simulink model "Pokus07_Display"  (Simulink 8.1)
settings: Solver=ode45  StartTime=0.0  StopTime=10.0  RelTol=1e-3
undefined symbols (not defined in the file): A, ARROW_DOWN, ARROW_LEFT, ARROW_RIGHT, ARROW_UP, ASTERISK, B, BACKSLASH, C, COLON, COMMA, CROSS, CURSOR, D, DOT, ending_column_index, ending_row_index, EQUAL, EXCLAMATION_MARK, F, framebuffer, G, GREATER_THAN, H, HEIGHT, hot, I, J, K, L, LEFT_PARENTHESES, LESS_THAN, M, MINUS, N, O, P, PERCENT, PLUS, POS_X, POS_Y, Q, QUESTION_MARK, QUOTE, R, RECTANGLE, RIGHT_PARENTHESES, S, SEMICOLON, SHARP, SLASH, SPACE, starting_column_index, starting_row_index, T, U, UNDERSCORE, V, W, WIDTH ... (+6)
libraries: dspmtrx3 x197, Common_Library x69, commutil2 x53, simulink_extras x1, dspsnks4 x1
(part 4 of 6)

== system Pokus07_Display/Character_Table/Characters(ARROW_DOWN..RECTANGLE)/Char_ARROW_LEFT ==
  Byte_01 : Constant  Value=char(2, ARROW_LEFT)  OutDataTypeStr=uint8
  Byte_02 : Constant  Value=char(3, ARROW_LEFT)  OutDataTypeStr=uint8
  Byte_03 : Constant  Value=char(4, ARROW_LEFT)  OutDataTypeStr=uint8
  Byte_04 : Constant  Value=char(5, ARROW_LEFT)  OutDataTypeStr=uint8
  Byte_05 : Constant  Value=char(6, ARROW_LEFT)  OutDataTypeStr=uint8
  Byte_06 : Constant  Value=char(7, ARROW_LEFT)  OutDataTypeStr=uint8
  Byte_07 : Constant  Value=char(8, ARROW_LEFT)  OutDataTypeStr=uint8
  Byte_1 : Constant  Value=char(1, ARROW_LEFT)  OutDataTypeStr=uint8
  Column_1(1B) : Outport
  Column_2(1B) : Outport  Port=2
  Column_3(1B) : Outport  Port=3
  Column_4(1B) : Outport  Port=4
  Column_5(1B) : Outport  Port=5
  Column_6(1B) : Outport  Port=6
  Column_7(1B) : Outport  Port=7
  Column_8(1B) : Outport  Port=8
  wires:
  Byte_05/1 -> Column_6(1B)/1
  Byte_04/1 -> Column_5(1B)/1
  Byte_01/1 -> Column_2(1B)/1
  Byte_07/1 -> Column_8(1B)/1
  Byte_03/1 -> Column_4(1B)/1
  Byte_06/1 -> Column_7(1B)/1
  Byte_1/1 -> Column_1(1B)/1
  Byte_02/1 -> Column_3(1B)/1

== system Pokus07_Display/Character_Table/Characters(ARROW_DOWN..RECTANGLE)/Char_ARROW_RIGHT ==
  Byte_01 : Constant  Value=char(2, ARROW_RIGHT)  OutDataTypeStr=uint8
  Byte_02 : Constant  Value=char(3, ARROW_RIGHT)  OutDataTypeStr=uint8
  Byte_03 : Constant  Value=char(4, ARROW_RIGHT)  OutDataTypeStr=uint8
  Byte_04 : Constant  Value=char(5, ARROW_RIGHT)  OutDataTypeStr=uint8
  Byte_05 : Constant  Value=char(6, ARROW_RIGHT)  OutDataTypeStr=uint8
  Byte_06 : Constant  Value=char(7, ARROW_RIGHT)  OutDataTypeStr=uint8
  Byte_07 : Constant  Value=char(8, ARROW_RIGHT)  OutDataTypeStr=uint8
  Byte_1 : Constant  Value=char(1, ARROW_RIGHT)  OutDataTypeStr=uint8
  Column_1(1B) : Outport
  Column_2(1B) : Outport  Port=2
  Column_3(1B) : Outport  Port=3
  Column_4(1B) : Outport  Port=4
  Column_5(1B) : Outport  Port=5
  Column_6(1B) : Outport  Port=6
  Column_7(1B) : Outport  Port=7
  Column_8(1B) : Outport  Port=8
  wires:
  Byte_05/1 -> Column_6(1B)/1
  Byte_04/1 -> Column_5(1B)/1
  Byte_01/1 -> Column_2(1B)/1
  Byte_07/1 -> Column_8(1B)/1
  Byte_03/1 -> Column_4(1B)/1
  Byte_06/1 -> Column_7(1B)/1
  Byte_1/1 -> Column_1(1B)/1
  Byte_02/1 -> Column_3(1B)/1

== system Pokus07_Display/Character_Table/Characters(ARROW_DOWN..RECTANGLE)/Char_COMMA ==
  Byte_01 : Constant  Value=char(2, COMMA)  OutDataTypeStr=uint8
  Byte_02 : Constant  Value=char(3, COMMA)  OutDataTypeStr=uint8
  Byte_03 : Constant  Value=char(4, COMMA)  OutDataTypeStr=uint8
  Byte_04 : Constant  Value=char(5, COMMA)  OutDataTypeStr=uint8
  Byte_05 : Constant  Value=char(6, COMMA)  OutDataTypeStr=uint8
  Byte_06 : Constant  Value=char(7, COMMA)  OutDataTypeStr=uint8
  Byte_07 : Constant  Value=char(8, COMMA)  OutDataTypeStr=uint8
  Byte_1 : Constant  Value=char(1, COMMA)  OutDataTypeStr=uint8
  Column_1(1B) : Outport
  Column_2(1B) : Outport  Port=2
  Column_3(1B) : Outport  Port=3
  Column_4(1B) : Outport  Port=4
  Column_5(1B) : Outport  Port=5
  Column_6(1B) : Outport  Port=6
  Column_7(1B) : Outport  Port=7
  Column_8(1B) : Outport  Port=8
  wires:
  Byte_05/1 -> Column_6(1B)/1
  Byte_04/1 -> Column_5(1B)/1
  Byte_01/1 -> Column_2(1B)/1
  Byte_07/1 -> Column_8(1B)/1
  Byte_03/1 -> Column_4(1B)/1
  Byte_06/1 -> Column_7(1B)/1
  Byte_1/1 -> Column_1(1B)/1
  Byte_02/1 -> Column_3(1B)/1

== system Pokus07_Display/Character_Table/Characters(ARROW_DOWN..RECTANGLE)/Char_CURSOR ==
  Byte_01 : Constant  Value=char(2, CURSOR)  OutDataTypeStr=uint8
  Byte_02 : Constant  Value=char(3, CURSOR)  OutDataTypeStr=uint8
  Byte_03 : Constant  Value=char(4, CURSOR)  OutDataTypeStr=uint8
  Byte_04 : Constant  Value=char(5, CURSOR)  OutDataTypeStr=uint8
  Byte_05 : Constant  Value=char(6, CURSOR)  OutDataTypeStr=uint8
  Byte_06 : Constant  Value=char(7, CURSOR)  OutDataTypeStr=uint8
  Byte_07 : Constant  Value=char(8, CURSOR)  OutDataTypeStr=uint8
  Byte_1 : Constant  Value=char(1, CURSOR)  OutDataTypeStr=uint8
  Column_1(1B) : Outport
  Column_2(1B) : Outport  Port=2
  Column_3(1B) : Outport  Port=3
  Column_4(1B) : Outport  Port=4
  Column_5(1B) : Outport  Port=5
  Column_6(1B) : Outport  Port=6
  Column_7(1B) : Outport  Port=7
  Column_8(1B) : Outport  Port=8
  wires:
  Byte_05/1 -> Column_6(1B)/1
  Byte_04/1 -> Column_5(1B)/1
  Byte_01/1 -> Column_2(1B)/1
  Byte_07/1 -> Column_8(1B)/1
  Byte_03/1 -> Column_4(1B)/1
  Byte_06/1 -> Column_7(1B)/1
  Byte_1/1 -> Column_1(1B)/1
  Byte_02/1 -> Column_3(1B)/1

== system Pokus07_Display/Character_Table/Characters(ARROW_DOWN..RECTANGLE)/Char_DOT ==
  Byte_01 : Constant  Value=char(2, DOT)  OutDataTypeStr=uint8
  Byte_02 : Constant  Value=char(3, DOT)  OutDataTypeStr=uint8
  Byte_03 : Constant  Value=char(4, DOT)  OutDataTypeStr=uint8
  Byte_04 : Constant  Value=char(5, DOT)  OutDataTypeStr=uint8
  Byte_05 : Constant  Value=char(6, DOT)  OutDataTypeStr=uint8
  Byte_06 : Constant  Value=char(7, DOT)  OutDataTypeStr=uint8
  Byte_07 : Constant  Value=char(8, DOT)  OutDataTypeStr=uint8
  Byte_1 : Constant  Value=char(1, DOT)  OutDataTypeStr=uint8
  Column_1(1B) : Outport
  Column_2(1B) : Outport  Port=2
  Column_3(1B) : Outport  Port=3
  Column_4(1B) : Outport  Port=4
  Column_5(1B) : Outport  Port=5
  Column_6(1B) : Outport  Port=6
  Column_7(1B) : Outport  Port=7
  Column_8(1B) : Outport  Port=8
  wires:
  Byte_05/1 -> Column_6(1B)/1
  Byte_04/1 -> Column_5(1B)/1
  Byte_01/1 -> Column_2(1B)/1
  Byte_07/1 -> Column_8(1B)/1
  Byte_03/1 -> Column_4(1B)/1
  Byte_06/1 -> Column_7(1B)/1
  Byte_1/1 -> Column_1(1B)/1
  Byte_02/1 -> Column_3(1B)/1

== system Pokus07_Display/Character_Table/Characters(ARROW_DOWN..RECTANGLE)/Char_EXCLAMATION_MARK ==
  Byte_01 : Constant  Value=char(2, EXCLAMATION_MARK)  OutDataTypeStr=uint8
  Byte_02 : Constant  Value=char(3, EXCLAMATION_MARK)  OutDataTypeStr=uint8
  Byte_03 : Constant  Value=char(4, EXCLAMATION_MARK)  OutDataTypeStr=uint8
  Byte_04 : Constant  Value=char(5, EXCLAMATION_MARK)  OutDataTypeStr=uint8
  Byte_05 : Constant  Value=char(6, EXCLAMATION_MARK)  OutDataTypeStr=uint8
  Byte_06 : Constant  Value=char(7, EXCLAMATION_MARK)  OutDataTypeStr=uint8
  Byte_07 : Constant  Value=char(8, EXCLAMATION_MARK)  OutDataTypeStr=uint8
  Byte_1 : Constant  Value=char(1, EXCLAMATION_MARK)  OutDataTypeStr=uint8
  Column_1(1B) : Outport
  Column_2(1B) : Outport  Port=2
  Column_3(1B) : Outport  Port=3
  Column_4(1B) : Outport  Port=4
  Column_5(1B) : Outport  Port=5
  Column_6(1B) : Outport  Port=6
  Column_7(1B) : Outport  Port=7
  Column_8(1B) : Outport  Port=8
  wires:
  Byte_05/1 -> Column_6(1B)/1
  Byte_04/1 -> Column_5(1B)/1
  Byte_01/1 -> Column_2(1B)/1
  Byte_07/1 -> Column_8(1B)/1
  Byte_03/1 -> Column_4(1B)/1
  Byte_06/1 -> Column_7(1B)/1
  Byte_1/1 -> Column_1(1B)/1
  Byte_02/1 -> Column_3(1B)/1

== system Pokus07_Display/Character_Table/Characters(ARROW_DOWN..RECTANGLE)/Char_LEFT_PARENTHESES ==
  Byte_01 : Constant  Value=char(2, LEFT_PARENTHESES)  OutDataTypeStr=uint8
  Byte_02 : Constant  Value=char(3, LEFT_PARENTHESES)  OutDataTypeStr=uint8
  Byte_03 : Constant  Value=char(4, LEFT_PARENTHESES)  OutDataTypeStr=uint8
  Byte_04 : Constant  Value=char(5, LEFT_PARENTHESES)  OutDataTypeStr=uint8
  Byte_05 : Constant  Value=char(6, LEFT_PARENTHESES)  OutDataTypeStr=uint8
  Byte_06 : Constant  Value=char(7, LEFT_PARENTHESES)  OutDataTypeStr=uint8
  Byte_07 : Constant  Value=char(8, LEFT_PARENTHESES)  OutDataTypeStr=uint8
  Byte_1 : Constant  Value=char(1, LEFT_PARENTHESES)  OutDataTypeStr=uint8
  Column_1(1B) : Outport
  Column_2(1B) : Outport  Port=2
  Column_3(1B) : Outport  Port=3
  Column_4(1B) : Outport  Port=4
  Column_5(1B) : Outport  Port=5
  Column_6(1B) : Outport  Port=6
  Column_7(1B) : Outport  Port=7
  Column_8(1B) : Outport  Port=8
  wires:
  Byte_05/1 -> Column_6(1B)/1
  Byte_04/1 -> Column_5(1B)/1
  Byte_01/1 -> Column_2(1B)/1
  Byte_07/1 -> Column_8(1B)/1
  Byte_03/1 -> Column_4(1B)/1
  Byte_06/1 -> Column_7(1B)/1
  Byte_1/1 -> Column_1(1B)/1
  Byte_02/1 -> Column_3(1B)/1

== system Pokus07_Display/Character_Table/Characters(ARROW_DOWN..RECTANGLE)/Char_PERCENT ==
  Byte_01 : Constant  Value=char(2, PERCENT)  OutDataTypeStr=uint8
  Byte_02 : Constant  Value=char(3, PERCENT)  OutDataTypeStr=uint8
  Byte_03 : Constant  Value=char(4, PERCENT)  OutDataTypeStr=uint8
  Byte_04 : Constant  Value=char(5, PERCENT)  OutDataTypeStr=uint8
  Byte_05 : Constant  Value=char(6, PERCENT)  OutDataTypeStr=uint8
  Byte_06 : Constant  Value=char(7, PERCENT)  OutDataTypeStr=uint8
  Byte_07 : Constant  Value=char(8, PERCENT)  OutDataTypeStr=uint8
  Byte_1 : Constant  Value=char(1, PERCENT)  OutDataTypeStr=uint8
  Column_1(1B) : Outport
  Column_2(1B) : Outport  Port=2
  Column_3(1B) : Outport  Port=3
  Column_4(1B) : Outport  Port=4
  Column_5(1B) : Outport  Port=5
  Column_6(1B) : Outport  Port=6
  Column_7(1B) : Outport  Port=7
  Column_8(1B) : Outport  Port=8
  wires:
  Byte_05/1 -> Column_6(1B)/1
  Byte_04/1 -> Column_5(1B)/1
  Byte_01/1 -> Column_2(1B)/1
  Byte_07/1 -> Column_8(1B)/1
  Byte_03/1 -> Column_4(1B)/1
  Byte_06/1 -> Column_7(1B)/1
  Byte_1/1 -> Column_1(1B)/1
  Byte_02/1 -> Column_3(1B)/1

== system Pokus07_Display/Character_Table/Characters(ARROW_DOWN..RECTANGLE)/Char_QUESTION_MARK ==
  Byte_01 : Constant  Value=char(2, QUESTION_MARK)  OutDataTypeStr=uint8
  Byte_02 : Constant  Value=char(3, QUESTION_MARK)  OutDataTypeStr=uint8
  Byte_03 : Constant  Value=char(4, QUESTION_MARK)  OutDataTypeStr=uint8
  Byte_04 : Constant  Value=char(5, QUESTION_MARK)  OutDataTypeStr=uint8
  Byte_05 : Constant  Value=char(6, QUESTION_MARK)  OutDataTypeStr=uint8
  Byte_06 : Constant  Value=char(7, QUESTION_MARK)  OutDataTypeStr=uint8
  Byte_07 : Constant  Value=char(8, QUESTION_MARK)  OutDataTypeStr=uint8
  Byte_1 : Constant  Value=char(1, QUESTION_MARK)  OutDataTypeStr=uint8
  Column_1(1B) : Outport
  Column_2(1B) : Outport  Port=2
  Column_3(1B) : Outport  Port=3
  Column_4(1B) : Outport  Port=4
  Column_5(1B) : Outport  Port=5
  Column_6(1B) : Outport  Port=6
  Column_7(1B) : Outport  Port=7
  Column_8(1B) : Outport  Port=8
  wires:
  Byte_05/1 -> Column_6(1B)/1
  Byte_04/1 -> Column_5(1B)/1
  Byte_01/1 -> Column_2(1B)/1
  Byte_07/1 -> Column_8(1B)/1
  Byte_03/1 -> Column_4(1B)/1
  Byte_06/1 -> Column_7(1B)/1
  Byte_1/1 -> Column_1(1B)/1
  Byte_02/1 -> Column_3(1B)/1

== system Pokus07_Display/Character_Table/Characters(ARROW_DOWN..RECTANGLE)/Char_QUOTE ==
  Byte_01 : Constant  Value=char(2, QUOTE)  OutDataTypeStr=uint8
  Byte_02 : Constant  Value=char(3, QUOTE)  OutDataTypeStr=uint8
  Byte_03 : Constant  Value=char(4, QUOTE)  OutDataTypeStr=uint8
  Byte_04 : Constant  Value=char(5, QUOTE)  OutDataTypeStr=uint8
  Byte_05 : Constant  Value=char(6, QUOTE)  OutDataTypeStr=uint8
  Byte_06 : Constant  Value=char(7, QUOTE)  OutDataTypeStr=uint8
  Byte_07 : Constant  Value=char(8, QUOTE)  OutDataTypeStr=uint8
  Byte_1 : Constant  Value=char(1, QUOTE)  OutDataTypeStr=uint8
  Column_1(1B) : Outport
  Column_2(1B) : Outport  Port=2
  Column_3(1B) : Outport  Port=3
  Column_4(1B) : Outport  Port=4
  Column_5(1B) : Outport  Port=5
  Column_6(1B) : Outport  Port=6
  Column_7(1B) : Outport  Port=7
  Column_8(1B) : Outport  Port=8
  wires:
  Byte_05/1 -> Column_6(1B)/1
  Byte_04/1 -> Column_5(1B)/1
  Byte_01/1 -> Column_2(1B)/1
  Byte_07/1 -> Column_8(1B)/1
  Byte_03/1 -> Column_4(1B)/1
  Byte_06/1 -> Column_7(1B)/1
  Byte_1/1 -> Column_1(1B)/1
  Byte_02/1 -> Column_3(1B)/1

== system Pokus07_Display/Character_Table/Characters(ARROW_DOWN..RECTANGLE)/Char_RECTANGLE ==
  Byte_01 : Constant  Value=char(2, RECTANGLE)  OutDataTypeStr=uint8
  Byte_02 : Constant  Value=char(3, RECTANGLE)  OutDataTypeStr=uint8
  Byte_03 : Constant  Value=char(4, RECTANGLE)  OutDataTypeStr=uint8
  Byte_04 : Constant  Value=char(5, RECTANGLE)  OutDataTypeStr=uint8
  Byte_05 : Constant  Value=char(6, RECTANGLE)  OutDataTypeStr=uint8
  Byte_06 : Constant  Value=char(7, RECTANGLE)  OutDataTypeStr=uint8
  Byte_07 : Constant  Value=char(8, RECTANGLE)  OutDataTypeStr=uint8
  Byte_1 : Constant  Value=char(1, RECTANGLE)  OutDataTypeStr=uint8
  Column_1(1B) : Outport
  Column_2(1B) : Outport  Port=2
  Column_3(1B) : Outport  Port=3
  Column_4(1B) : Outport  Port=4
  Column_5(1B) : Outport  Port=5
  Column_6(1B) : Outport  Port=6
  Column_7(1B) : Outport  Port=7
  Column_8(1B) : Outport  Port=8
  wires:
  Byte_05/1 -> Column_6(1B)/1
  Byte_04/1 -> Column_5(1B)/1
  Byte_01/1 -> Column_2(1B)/1
  Byte_07/1 -> Column_8(1B)/1
  Byte_03/1 -> Column_4(1B)/1
  Byte_06/1 -> Column_7(1B)/1
  Byte_1/1 -> Column_1(1B)/1
  Byte_02/1 -> Column_3(1B)/1

== system Pokus07_Display/Character_Table/Characters(ARROW_DOWN..RECTANGLE)/Char_RIGHT_PARENTHESES ==
  Byte_01 : Constant  Value=char(2, RIGHT_PARENTHESES)  OutDataTypeStr=uint8
  Byte_02 : Constant  Value=char(3, RIGHT_PARENTHESES)  OutDataTypeStr=uint8
  Byte_03 : Constant  Value=char(4, RIGHT_PARENTHESES)  OutDataTypeStr=uint8
  Byte_04 : Constant  Value=char(5, RIGHT_PARENTHESES)  OutDataTypeStr=uint8
  Byte_05 : Constant  Value=char(6, RIGHT_PARENTHESES)  OutDataTypeStr=uint8
  Byte_06 : Constant  Value=char(7, RIGHT_PARENTHESES)  OutDataTypeStr=uint8
  Byte_07 : Constant  Value=char(8, RIGHT_PARENTHESES)  OutDataTypeStr=uint8
  Byte_1 : Constant  Value=char(1, RIGHT_PARENTHESES)  OutDataTypeStr=uint8
  Column_1(1B) : Outport
  Column_2(1B) : Outport  Port=2
  Column_3(1B) : Outport  Port=3
  Column_4(1B) : Outport  Port=4
  Column_5(1B) : Outport  Port=5
  Column_6(1B) : Outport  Port=6
  Column_7(1B) : Outport  Port=7
  Column_8(1B) : Outport  Port=8
  wires:
  Byte_05/1 -> Column_6(1B)/1
  Byte_04/1 -> Column_5(1B)/1
  Byte_01/1 -> Column_2(1B)/1
  Byte_07/1 -> Column_8(1B)/1
  Byte_03/1 -> Column_4(1B)/1
  Byte_06/1 -> Column_7(1B)/1
  Byte_1/1 -> Column_1(1B)/1
  Byte_02/1 -> Column_3(1B)/1

== system Pokus07_Display/Character_Table/Characters(ARROW_DOWN..RECTANGLE)/Char_SHARP ==
  Byte_01 : Constant  Value=char(2, SHARP)  OutDataTypeStr=uint8
  Byte_02 : Constant  Value=char(3, SHARP)  OutDataTypeStr=uint8
  Byte_03 : Constant  Value=char(4, SHARP)  OutDataTypeStr=uint8
  Byte_04 : Constant  Value=char(5, SHARP)  OutDataTypeStr=uint8
  Byte_05 : Constant  Value=char(6, SHARP)  OutDataTypeStr=uint8
  Byte_06 : Constant  Value=char(7, SHARP)  OutDataTypeStr=uint8
  Byte_07 : Constant  Value=char(8, SHARP)  OutDataTypeStr=uint8
  Byte_1 : Constant  Value=char(1, SHARP)  OutDataTypeStr=uint8
  Column_1(1B) : Outport
  Column_2(1B) : Outport  Port=2
  Column_3(1B) : Outport  Port=3
  Column_4(1B) : Outport  Port=4
  Column_5(1B) : Outport  Port=5
  Column_6(1B) : Outport  Port=6
  Column_7(1B) : Outport  Port=7
  Column_8(1B) : Outport  Port=8
  wires:
  Byte_05/1 -> Column_6(1B)/1
  Byte_04/1 -> Column_5(1B)/1
  Byte_01/1 -> Column_2(1B)/1
  Byte_07/1 -> Column_8(1B)/1
  Byte_03/1 -> Column_4(1B)/1
  Byte_06/1 -> Column_7(1B)/1
  Byte_1/1 -> Column_1(1B)/1
  Byte_02/1 -> Column_3(1B)/1

== system Pokus07_Display/Character_Table/Characters(ARROW_DOWN..RECTANGLE)/Char_SPACE ==
  Byte_01 : Constant  Value=char(2, SPACE)  OutDataTypeStr=uint8
  Byte_02 : Constant  Value=char(3, SPACE)  OutDataTypeStr=uint8
  Byte_03 : Constant  Value=char(4, SPACE)  OutDataTypeStr=uint8
  Byte_04 : Constant  Value=char(5, SPACE)  OutDataTypeStr=uint8
  Byte_05 : Constant  Value=char(6, SPACE)  OutDataTypeStr=uint8
  Byte_06 : Constant  Value=char(7, SPACE)  OutDataTypeStr=uint8
  Byte_07 : Constant  Value=char(8, SPACE)  OutDataTypeStr=uint8
  Byte_1 : Constant  Value=char(1, SPACE)  OutDataTypeStr=uint8
  Column_1(1B) : Outport
  Column_2(1B) : Outport  Port=2
  Column_3(1B) : Outport  Port=3
  Column_4(1B) : Outport  Port=4
  Column_5(1B) : Outport  Port=5
  Column_6(1B) : Outport  Port=6
  Column_7(1B) : Outport  Port=7
  Column_8(1B) : Outport  Port=8
  wires:
  Byte_05/1 -> Column_6(1B)/1
  Byte_04/1 -> Column_5(1B)/1
  Byte_01/1 -> Column_2(1B)/1
  Byte_07/1 -> Column_8(1B)/1
  Byte_03/1 -> Column_4(1B)/1
  Byte_06/1 -> Column_7(1B)/1
  Byte_1/1 -> Column_1(1B)/1
  Byte_02/1 -> Column_3(1B)/1

== system Pokus07_Display/Character_Table/Characters(ARROW_DOWN..RECTANGLE)/Char_UNDERSCORE ==
  Byte_01 : Constant  Value=char(2, UNDERSCORE)  OutDataTypeStr=uint8
  Byte_02 : Constant  Value=char(3, UNDERSCORE)  OutDataTypeStr=uint8
  Byte_03 : Constant  Value=char(4, UNDERSCORE)  OutDataTypeStr=uint8
  Byte_04 : Constant  Value=char(5, UNDERSCORE)  OutDataTypeStr=uint8
  Byte_05 : Constant  Value=char(6, UNDERSCORE)  OutDataTypeStr=uint8
  Byte_06 : Constant  Value=char(7, UNDERSCORE)  OutDataTypeStr=uint8
  Byte_07 : Constant  Value=char(8, UNDERSCORE)  OutDataTypeStr=uint8
  Byte_1 : Constant  Value=char(1, UNDERSCORE)  OutDataTypeStr=uint8
  Column_1(1B) : Outport
  Column_2(1B) : Outport  Port=2
  Column_3(1B) : Outport  Port=3
  Column_4(1B) : Outport  Port=4
  Column_5(1B) : Outport  Port=5
  Column_6(1B) : Outport  Port=6
  Column_7(1B) : Outport  Port=7
  Column_8(1B) : Outport  Port=8
  wires:
  Byte_05/1 -> Column_6(1B)/1
  Byte_04/1 -> Column_5(1B)/1
  Byte_01/1 -> Column_2(1B)/1
  Byte_07/1 -> Column_8(1B)/1
  Byte_03/1 -> Column_4(1B)/1
  Byte_06/1 -> Column_7(1B)/1
  Byte_1/1 -> Column_1(1B)/1
  Byte_02/1 -> Column_3(1B)/1

== system Pokus07_Display/Character_Table/Characters(ARROW_DOWN..RECTANGLE)1/Char_ARROW_DOWN ==
  Byte_01 : Constant  Value=char(2, ARROW_DOWN)  OutDataTypeStr=uint8
  Byte_02 : Constant  Value=char(3, ARROW_DOWN)  OutDataTypeStr=uint8
  Byte_03 : Constant  Value=char(4, ARROW_DOWN)  OutDataTypeStr=uint8
  Byte_04 : Constant  Value=char(5, ARROW_DOWN)  OutDataTypeStr=uint8
  Byte_05 : Constant  Value=char(6, ARROW_DOWN)  OutDataTypeStr=uint8
  Byte_06 : Constant  Value=char(7, ARROW_DOWN)  OutDataTypeStr=uint8
  Byte_07 : Constant  Value=char(8, ARROW_DOWN)  OutDataTypeStr=uint8
  Byte_1 : Constant  Value=char(1, ARROW_DOWN)  OutDataTypeStr=uint8
  Column_1(1B) : Outport
  Column_2(1B) : Outport  Port=2
  Column_3(1B) : Outport  Port=3
  Column_4(1B) : Outport  Port=4
  Column_5(1B) : Outport  Port=5
  Column_6(1B) : Outport  Port=6
  Column_7(1B) : Outport  Port=7
  Column_8(1B) : Outport  Port=8
  wires:
  Byte_05/1 -> Column_6(1B)/1
  Byte_04/1 -> Column_5(1B)/1
  Byte_01/1 -> Column_2(1B)/1
  Byte_07/1 -> Column_8(1B)/1
  Byte_03/1 -> Column_4(1B)/1
  Byte_06/1 -> Column_7(1B)/1
  Byte_1/1 -> Column_1(1B)/1
  Byte_02/1 -> Column_3(1B)/1

== system Pokus07_Display/Character_Table/Characters(ARROW_DOWN..RECTANGLE)1/Char_ARROW_LEFT ==
  Byte_01 : Constant  Value=char(2, ARROW_LEFT)  OutDataTypeStr=uint8
  Byte_02 : Constant  Value=char(3, ARROW_LEFT)  OutDataTypeStr=uint8
  Byte_03 : Constant  Value=char(4, ARROW_LEFT)  OutDataTypeStr=uint8
  Byte_04 : Constant  Value=char(5, ARROW_LEFT)  OutDataTypeStr=uint8
  Byte_05 : Constant  Value=char(6, ARROW_LEFT)  OutDataTypeStr=uint8
  Byte_06 : Constant  Value=char(7, ARROW_LEFT)  OutDataTypeStr=uint8
  Byte_07 : Constant  Value=char(8, ARROW_LEFT)  OutDataTypeStr=uint8
  Byte_1 : Constant  Value=char(1, ARROW_LEFT)  OutDataTypeStr=uint8
  Column_1(1B) : Outport
  Column_2(1B) : Outport  Port=2
  Column_3(1B) : Outport  Port=3
  Column_4(1B) : Outport  Port=4
  Column_5(1B) : Outport  Port=5
  Column_6(1B) : Outport  Port=6
  Column_7(1B) : Outport  Port=7
  Column_8(1B) : Outport  Port=8
  wires:
  Byte_05/1 -> Column_6(1B)/1
  Byte_04/1 -> Column_5(1B)/1
  Byte_01/1 -> Column_2(1B)/1
  Byte_07/1 -> Column_8(1B)/1
  Byte_03/1 -> Column_4(1B)/1
  Byte_06/1 -> Column_7(1B)/1
  Byte_1/1 -> Column_1(1B)/1
  Byte_02/1 -> Column_3(1B)/1

== system Pokus07_Display/Character_Table/Characters(ARROW_DOWN..RECTANGLE)1/Char_ARROW_RIGHT ==
  Byte_01 : Constant  Value=char(2, ARROW_RIGHT)  OutDataTypeStr=uint8
  Byte_02 : Constant  Value=char(3, ARROW_RIGHT)  OutDataTypeStr=uint8
  Byte_03 : Constant  Value=char(4, ARROW_RIGHT)  OutDataTypeStr=uint8
  Byte_04 : Constant  Value=char(5, ARROW_RIGHT)  OutDataTypeStr=uint8
  Byte_05 : Constant  Value=char(6, ARROW_RIGHT)  OutDataTypeStr=uint8
  Byte_06 : Constant  Value=char(7, ARROW_RIGHT)  OutDataTypeStr=uint8
  Byte_07 : Constant  Value=char(8, ARROW_RIGHT)  OutDataTypeStr=uint8
  Byte_1 : Constant  Value=char(1, ARROW_RIGHT)  OutDataTypeStr=uint8
  Column_1(1B) : Outport
  Column_2(1B) : Outport  Port=2
  Column_3(1B) : Outport  Port=3
  Column_4(1B) : Outport  Port=4
  Column_5(1B) : Outport  Port=5
  Column_6(1B) : Outport  Port=6
  Column_7(1B) : Outport  Port=7
  Column_8(1B) : Outport  Port=8
  wires:
  Byte_05/1 -> Column_6(1B)/1
  Byte_04/1 -> Column_5(1B)/1
  Byte_01/1 -> Column_2(1B)/1
  Byte_07/1 -> Column_8(1B)/1
  Byte_03/1 -> Column_4(1B)/1
  Byte_06/1 -> Column_7(1B)/1
  Byte_1/1 -> Column_1(1B)/1
  Byte_02/1 -> Column_3(1B)/1

== system Pokus07_Display/Character_Table/Characters(ARROW_DOWN..RECTANGLE)1/Char_COMMA ==
  Byte_01 : Constant  Value=char(2, COMMA)  OutDataTypeStr=uint8
  Byte_02 : Constant  Value=char(3, COMMA)  OutDataTypeStr=uint8
  Byte_03 : Constant  Value=char(4, COMMA)  OutDataTypeStr=uint8
  Byte_04 : Constant  Value=char(5, COMMA)  OutDataTypeStr=uint8
  Byte_05 : Constant  Value=char(6, COMMA)  OutDataTypeStr=uint8
  Byte_06 : Constant  Value=char(7, COMMA)  OutDataTypeStr=uint8
  Byte_07 : Constant  Value=char(8, COMMA)  OutDataTypeStr=uint8
  Byte_1 : Constant  Value=char(1, COMMA)  OutDataTypeStr=uint8
  Column_1(1B) : Outport
  Column_2(1B) : Outport  Port=2
  Column_3(1B) : Outport  Port=3
  Column_4(1B) : Outport  Port=4
  Column_5(1B) : Outport  Port=5
  Column_6(1B) : Outport  Port=6
  Column_7(1B) : Outport  Port=7
  Column_8(1B) : Outport  Port=8
  wires:
  Byte_05/1 -> Column_6(1B)/1
  Byte_04/1 -> Column_5(1B)/1
  Byte_01/1 -> Column_2(1B)/1
  Byte_07/1 -> Column_8(1B)/1
  Byte_03/1 -> Column_4(1B)/1
  Byte_06/1 -> Column_7(1B)/1
  Byte_1/1 -> Column_1(1B)/1
  Byte_02/1 -> Column_3(1B)/1

== system Pokus07_Display/Character_Table/Characters(ARROW_DOWN..RECTANGLE)1/Char_CURSOR ==
  Byte_01 : Constant  Value=char(2, CURSOR)  OutDataTypeStr=uint8
  Byte_02 : Constant  Value=char(3, CURSOR)  OutDataTypeStr=uint8
  Byte_03 : Constant  Value=char(4, CURSOR)  OutDataTypeStr=uint8
  Byte_04 : Constant  Value=char(5, CURSOR)  OutDataTypeStr=uint8
  Byte_05 : Constant  Value=char(6, CURSOR)  OutDataTypeStr=uint8
  Byte_06 : Constant  Value=char(7, CURSOR)  OutDataTypeStr=uint8
  Byte_07 : Constant  Value=char(8, CURSOR)  OutDataTypeStr=uint8
  Byte_1 : Constant  Value=char(1, CURSOR)  OutDataTypeStr=uint8
  Column_1(1B) : Outport
  Column_2(1B) : Outport  Port=2
  Column_3(1B) : Outport  Port=3
  Column_4(1B) : Outport  Port=4
  Column_5(1B) : Outport  Port=5
  Column_6(1B) : Outport  Port=6
  Column_7(1B) : Outport  Port=7
  Column_8(1B) : Outport  Port=8
  wires:
  Byte_05/1 -> Column_6(1B)/1
  Byte_04/1 -> Column_5(1B)/1
  Byte_01/1 -> Column_2(1B)/1
  Byte_07/1 -> Column_8(1B)/1
  Byte_03/1 -> Column_4(1B)/1
  Byte_06/1 -> Column_7(1B)/1
  Byte_1/1 -> Column_1(1B)/1
  Byte_02/1 -> Column_3(1B)/1

== system Pokus07_Display/Character_Table/Characters(ARROW_DOWN..RECTANGLE)1/Char_DOT ==
  Byte_01 : Constant  Value=char(2, DOT)  OutDataTypeStr=uint8
  Byte_02 : Constant  Value=char(3, DOT)  OutDataTypeStr=uint8
  Byte_03 : Constant  Value=char(4, DOT)  OutDataTypeStr=uint8
  Byte_04 : Constant  Value=char(5, DOT)  OutDataTypeStr=uint8
  Byte_05 : Constant  Value=char(6, DOT)  OutDataTypeStr=uint8
  Byte_06 : Constant  Value=char(7, DOT)  OutDataTypeStr=uint8
  Byte_07 : Constant  Value=char(8, DOT)  OutDataTypeStr=uint8
  Byte_1 : Constant  Value=char(1, DOT)  OutDataTypeStr=uint8
  Column_1(1B) : Outport
  Column_2(1B) : Outport  Port=2
  Column_3(1B) : Outport  Port=3
  Column_4(1B) : Outport  Port=4
  Column_5(1B) : Outport  Port=5
  Column_6(1B) : Outport  Port=6
  Column_7(1B) : Outport  Port=7
  Column_8(1B) : Outport  Port=8
  wires:
  Byte_05/1 -> Column_6(1B)/1
  Byte_04/1 -> Column_5(1B)/1
  Byte_01/1 -> Column_2(1B)/1
  Byte_07/1 -> Column_8(1B)/1
  Byte_03/1 -> Column_4(1B)/1
  Byte_06/1 -> Column_7(1B)/1
  Byte_1/1 -> Column_1(1B)/1
  Byte_02/1 -> Column_3(1B)/1

== system Pokus07_Display/Character_Table/Characters(ARROW_DOWN..RECTANGLE)1/Char_EXCLAMATION_MARK ==
  Byte_01 : Constant  Value=char(2, EXCLAMATION_MARK)  OutDataTypeStr=uint8
  Byte_02 : Constant  Value=char(3, EXCLAMATION_MARK)  OutDataTypeStr=uint8
  Byte_03 : Constant  Value=char(4, EXCLAMATION_MARK)  OutDataTypeStr=uint8
  Byte_04 : Constant  Value=char(5, EXCLAMATION_MARK)  OutDataTypeStr=uint8
  Byte_05 : Constant  Value=char(6, EXCLAMATION_MARK)  OutDataTypeStr=uint8
  Byte_06 : Constant  Value=char(7, EXCLAMATION_MARK)  OutDataTypeStr=uint8
  Byte_07 : Constant  Value=char(8, EXCLAMATION_MARK)  OutDataTypeStr=uint8
  Byte_1 : Constant  Value=char(1, EXCLAMATION_MARK)  OutDataTypeStr=uint8
  Column_1(1B) : Outport
  Column_2(1B) : Outport  Port=2
  Column_3(1B) : Outport  Port=3
  Column_4(1B) : Outport  Port=4
  Column_5(1B) : Outport  Port=5
  Column_6(1B) : Outport  Port=6
  Column_7(1B) : Outport  Port=7
  Column_8(1B) : Outport  Port=8
  wires:
  Byte_05/1 -> Column_6(1B)/1
  Byte_04/1 -> Column_5(1B)/1
  Byte_01/1 -> Column_2(1B)/1
  Byte_07/1 -> Column_8(1B)/1
  Byte_03/1 -> Column_4(1B)/1
  Byte_06/1 -> Column_7(1B)/1
  Byte_1/1 -> Column_1(1B)/1
  Byte_02/1 -> Column_3(1B)/1

== system Pokus07_Display/Character_Table/Characters(ARROW_DOWN..RECTANGLE)1/Char_LEFT_PARENTHESES ==
  Byte_01 : Constant  Value=char(2, LEFT_PARENTHESES)  OutDataTypeStr=uint8
  Byte_02 : Constant  Value=char(3, LEFT_PARENTHESES)  OutDataTypeStr=uint8
  Byte_03 : Constant  Value=char(4, LEFT_PARENTHESES)  OutDataTypeStr=uint8
  Byte_04 : Constant  Value=char(5, LEFT_PARENTHESES)  OutDataTypeStr=uint8
  Byte_05 : Constant  Value=char(6, LEFT_PARENTHESES)  OutDataTypeStr=uint8
  Byte_06 : Constant  Value=char(7, LEFT_PARENTHESES)  OutDataTypeStr=uint8
  Byte_07 : Constant  Value=char(8, LEFT_PARENTHESES)  OutDataTypeStr=uint8
  Byte_1 : Constant  Value=char(1, LEFT_PARENTHESES)  OutDataTypeStr=uint8
  Column_1(1B) : Outport
  Column_2(1B) : Outport  Port=2
  Column_3(1B) : Outport  Port=3
  Column_4(1B) : Outport  Port=4
  Column_5(1B) : Outport  Port=5
  Column_6(1B) : Outport  Port=6
  Column_7(1B) : Outport  Port=7
  Column_8(1B) : Outport  Port=8
  wires:
  Byte_05/1 -> Column_6(1B)/1
  Byte_04/1 -> Column_5(1B)/1
  Byte_01/1 -> Column_2(1B)/1
  Byte_07/1 -> Column_8(1B)/1
  Byte_03/1 -> Column_4(1B)/1
  Byte_06/1 -> Column_7(1B)/1
  Byte_1/1 -> Column_1(1B)/1
  Byte_02/1 -> Column_3(1B)/1

== system Pokus07_Display/Character_Table/Characters(ARROW_DOWN..RECTANGLE)1/Char_PERCENT ==
  Byte_01 : Constant  Value=char(2, PERCENT)  OutDataTypeStr=uint8
  Byte_02 : Constant  Value=char(3, PERCENT)  OutDataTypeStr=uint8
  Byte_03 : Constant  Value=char(4, PERCENT)  OutDataTypeStr=uint8
  Byte_04 : Constant  Value=char(5, PERCENT)  OutDataTypeStr=uint8
  Byte_05 : Constant  Value=char(6, PERCENT)  OutDataTypeStr=uint8
  Byte_06 : Constant  Value=char(7, PERCENT)  OutDataTypeStr=uint8
  Byte_07 : Constant  Value=char(8, PERCENT)  OutDataTypeStr=uint8
  Byte_1 : Constant  Value=char(1, PERCENT)  OutDataTypeStr=uint8
  Column_1(1B) : Outport
  Column_2(1B) : Outport  Port=2
  Column_3(1B) : Outport  Port=3
  Column_4(1B) : Outport  Port=4
  Column_5(1B) : Outport  Port=5
  Column_6(1B) : Outport  Port=6
  Column_7(1B) : Outport  Port=7
  Column_8(1B) : Outport  Port=8
  wires:
  Byte_05/1 -> Column_6(1B)/1
  Byte_04/1 -> Column_5(1B)/1
  Byte_01/1 -> Column_2(1B)/1
  Byte_07/1 -> Column_8(1B)/1
  Byte_03/1 -> Column_4(1B)/1
  Byte_06/1 -> Column_7(1B)/1
  Byte_1/1 -> Column_1(1B)/1
  Byte_02/1 -> Column_3(1B)/1

== system Pokus07_Display/Character_Table/Characters(ARROW_DOWN..RECTANGLE)1/Char_QUESTION_MARK ==
  Byte_01 : Constant  Value=char(2, QUESTION_MARK)  OutDataTypeStr=uint8
  Byte_02 : Constant  Value=char(3, QUESTION_MARK)  OutDataTypeStr=uint8
  Byte_03 : Constant  Value=char(4, QUESTION_MARK)  OutDataTypeStr=uint8
  Byte_04 : Constant  Value=char(5, QUESTION_MARK)  OutDataTypeStr=uint8
  Byte_05 : Constant  Value=char(6, QUESTION_MARK)  OutDataTypeStr=uint8
  Byte_06 : Constant  Value=char(7, QUESTION_MARK)  OutDataTypeStr=uint8
  Byte_07 : Constant  Value=char(8, QUESTION_MARK)  OutDataTypeStr=uint8
  Byte_1 : Constant  Value=char(1, QUESTION_MARK)  OutDataTypeStr=uint8
  Column_1(1B) : Outport
  Column_2(1B) : Outport  Port=2
  Column_3(1B) : Outport  Port=3
  Column_4(1B) : Outport  Port=4
  Column_5(1B) : Outport  Port=5
  Column_6(1B) : Outport  Port=6
  Column_7(1B) : Outport  Port=7
  Column_8(1B) : Outport  Port=8
  wires:
  Byte_05/1 -> Column_6(1B)/1
  Byte_04/1 -> Column_5(1B)/1
  Byte_01/1 -> Column_2(1B)/1
  Byte_07/1 -> Column_8(1B)/1
  Byte_03/1 -> Column_4(1B)/1
  Byte_06/1 -> Column_7(1B)/1
  Byte_1/1 -> Column_1(1B)/1
  Byte_02/1 -> Column_3(1B)/1

== system Pokus07_Display/Character_Table/Characters(ARROW_DOWN..RECTANGLE)1/Char_QUOTE ==
  Byte_01 : Constant  Value=char(2, QUOTE)  OutDataTypeStr=uint8
  Byte_02 : Constant  Value=char(3, QUOTE)  OutDataTypeStr=uint8
  Byte_03 : Constant  Value=char(4, QUOTE)  OutDataTypeStr=uint8
  Byte_04 : Constant  Value=char(5, QUOTE)  OutDataTypeStr=uint8
  Byte_05 : Constant  Value=char(6, QUOTE)  OutDataTypeStr=uint8
  Byte_06 : Constant  Value=char(7, QUOTE)  OutDataTypeStr=uint8
  Byte_07 : Constant  Value=char(8, QUOTE)  OutDataTypeStr=uint8
  Byte_1 : Constant  Value=char(1, QUOTE)  OutDataTypeStr=uint8
  Column_1(1B) : Outport
  Column_2(1B) : Outport  Port=2
  Column_3(1B) : Outport  Port=3
  Column_4(1B) : Outport  Port=4
  Column_5(1B) : Outport  Port=5
  Column_6(1B) : Outport  Port=6
  Column_7(1B) : Outport  Port=7
  Column_8(1B) : Outport  Port=8
  wires:
  Byte_05/1 -> Column_6(1B)/1
  Byte_04/1 -> Column_5(1B)/1
  Byte_01/1 -> Column_2(1B)/1
  Byte_07/1 -> Column_8(1B)/1
  Byte_03/1 -> Column_4(1B)/1
  Byte_06/1 -> Column_7(1B)/1
  Byte_1/1 -> Column_1(1B)/1
  Byte_02/1 -> Column_3(1B)/1

== system Pokus07_Display/Character_Table/Characters(ARROW_DOWN..RECTANGLE)1/Char_RECTANGLE ==
  Byte_01 : Constant  Value=char(2, RECTANGLE)  OutDataTypeStr=uint8
  Byte_02 : Constant  Value=char(3, RECTANGLE)  OutDataTypeStr=uint8
  Byte_03 : Constant  Value=char(4, RECTANGLE)  OutDataTypeStr=uint8
  Byte_04 : Constant  Value=char(5, RECTANGLE)  OutDataTypeStr=uint8
  Byte_05 : Constant  Value=char(6, RECTANGLE)  OutDataTypeStr=uint8
  Byte_06 : Constant  Value=char(7, RECTANGLE)  OutDataTypeStr=uint8
  Byte_07 : Constant  Value=char(8, RECTANGLE)  OutDataTypeStr=uint8
  Byte_1 : Constant  Value=char(1, RECTANGLE)  OutDataTypeStr=uint8
  Column_1(1B) : Outport
  Column_2(1B) : Outport  Port=2
  Column_3(1B) : Outport  Port=3
  Column_4(1B) : Outport  Port=4
  Column_5(1B) : Outport  Port=5
  Column_6(1B) : Outport  Port=6
  Column_7(1B) : Outport  Port=7
  Column_8(1B) : Outport  Port=8
  wires:
  Byte_05/1 -> Column_6(1B)/1
  Byte_04/1 -> Column_5(1B)/1
  Byte_01/1 -> Column_2(1B)/1
  Byte_07/1 -> Column_8(1B)/1
  Byte_03/1 -> Column_4(1B)/1
  Byte_06/1 -> Column_7(1B)/1
  Byte_1/1 -> Column_1(1B)/1
  Byte_02/1 -> Column_3(1B)/1

== system Pokus07_Display/Character_Table/Characters(ARROW_DOWN..RECTANGLE)1/Char_RIGHT_PARENTHESES ==
  Byte_01 : Constant  Value=char(2, RIGHT_PARENTHESES)  OutDataTypeStr=uint8
  Byte_02 : Constant  Value=char(3, RIGHT_PARENTHESES)  OutDataTypeStr=uint8
  Byte_03 : Constant  Value=char(4, RIGHT_PARENTHESES)  OutDataTypeStr=uint8
  Byte_04 : Constant  Value=char(5, RIGHT_PARENTHESES)  OutDataTypeStr=uint8
  Byte_05 : Constant  Value=char(6, RIGHT_PARENTHESES)  OutDataTypeStr=uint8
  Byte_06 : Constant  Value=char(7, RIGHT_PARENTHESES)  OutDataTypeStr=uint8
  Byte_07 : Constant  Value=char(8, RIGHT_PARENTHESES)  OutDataTypeStr=uint8
  Byte_1 : Constant  Value=char(1, RIGHT_PARENTHESES)  OutDataTypeStr=uint8
  Column_1(1B) : Outport
  Column_2(1B) : Outport  Port=2
  Column_3(1B) : Outport  Port=3
  Column_4(1B) : Outport  Port=4
  Column_5(1B) : Outport  Port=5
  Column_6(1B) : Outport  Port=6
  Column_7(1B) : Outport  Port=7
  Column_8(1B) : Outport  Port=8
  wires:
  Byte_05/1 -> Column_6(1B)/1
  Byte_04/1 -> Column_5(1B)/1
  Byte_01/1 -> Column_2(1B)/1
  Byte_07/1 -> Column_8(1B)/1
  Byte_03/1 -> Column_4(1B)/1
  Byte_06/1 -> Column_7(1B)/1
  Byte_1/1 -> Column_1(1B)/1
  Byte_02/1 -> Column_3(1B)/1

== system Pokus07_Display/Character_Table/Characters(ARROW_DOWN..RECTANGLE)1/Char_SHARP ==
  Byte_01 : Constant  Value=char(2, SHARP)  OutDataTypeStr=uint8
  Byte_02 : Constant  Value=char(3, SHARP)  OutDataTypeStr=uint8
  Byte_03 : Constant  Value=char(4, SHARP)  OutDataTypeStr=uint8
  Byte_04 : Constant  Value=char(5, SHARP)  OutDataTypeStr=uint8
  Byte_05 : Constant  Value=char(6, SHARP)  OutDataTypeStr=uint8
  Byte_06 : Constant  Value=char(7, SHARP)  OutDataTypeStr=uint8
  Byte_07 : Constant  Value=char(8, SHARP)  OutDataTypeStr=uint8
  Byte_1 : Constant  Value=char(1, SHARP)  OutDataTypeStr=uint8
  Column_1(1B) : Outport
  Column_2(1B) : Outport  Port=2
  Column_3(1B) : Outport  Port=3
  Column_4(1B) : Outport  Port=4
  Column_5(1B) : Outport  Port=5
  Column_6(1B) : Outport  Port=6
  Column_7(1B) : Outport  Port=7
  Column_8(1B) : Outport  Port=8
  wires:
  Byte_05/1 -> Column_6(1B)/1
  Byte_04/1 -> Column_5(1B)/1
  Byte_01/1 -> Column_2(1B)/1
  Byte_07/1 -> Column_8(1B)/1
  Byte_03/1 -> Column_4(1B)/1
  Byte_06/1 -> Column_7(1B)/1
  Byte_1/1 -> Column_1(1B)/1
  Byte_02/1 -> Column_3(1B)/1

== system Pokus07_Display/Character_Table/Characters(ARROW_DOWN..RECTANGLE)1/Char_SPACE ==
  Byte_01 : Constant  Value=char(2, SPACE)  OutDataTypeStr=uint8
  Byte_02 : Constant  Value=char(3, SPACE)  OutDataTypeStr=uint8
  Byte_03 : Constant  Value=char(4, SPACE)  OutDataTypeStr=uint8
  Byte_04 : Constant  Value=char(5, SPACE)  OutDataTypeStr=uint8
  Byte_05 : Constant  Value=char(6, SPACE)  OutDataTypeStr=uint8
  Byte_06 : Constant  Value=char(7, SPACE)  OutDataTypeStr=uint8
  Byte_07 : Constant  Value=char(8, SPACE)  OutDataTypeStr=uint8
  Byte_1 : Constant  Value=char(1, SPACE)  OutDataTypeStr=uint8
  Column_1(1B) : Outport
  Column_2(1B) : Outport  Port=2
  Column_3(1B) : Outport  Port=3
  Column_4(1B) : Outport  Port=4
  Column_5(1B) : Outport  Port=5
  Column_6(1B) : Outport  Port=6
  Column_7(1B) : Outport  Port=7
  Column_8(1B) : Outport  Port=8
  wires:
  Byte_05/1 -> Column_6(1B)/1
  Byte_04/1 -> Column_5(1B)/1
  Byte_01/1 -> Column_2(1B)/1
  Byte_07/1 -> Column_8(1B)/1
  Byte_03/1 -> Column_4(1B)/1
  Byte_06/1 -> Column_7(1B)/1
  Byte_1/1 -> Column_1(1B)/1
  Byte_02/1 -> Column_3(1B)/1

== system Pokus07_Display/Character_Table/Characters(ARROW_DOWN..RECTANGLE)1/Char_UNDERSCORE ==
  Byte_01 : Constant  Value=char(2, UNDERSCORE)  OutDataTypeStr=uint8
  Byte_02 : Constant  Value=char(3, UNDERSCORE)  OutDataTypeStr=uint8
  Byte_03 : Constant  Value=char(4, UNDERSCORE)  OutDataTypeStr=uint8
  Byte_04 : Constant  Value=char(5, UNDERSCORE)  OutDataTypeStr=uint8
  Byte_05 : Constant  Value=char(6, UNDERSCORE)  OutDataTypeStr=uint8
  Byte_06 : Constant  Value=char(7, UNDERSCORE)  OutDataTypeStr=uint8
  Byte_07 : Constant  Value=char(8, UNDERSCORE)  OutDataTypeStr=uint8
  Byte_1 : Constant  Value=char(1, UNDERSCORE)  OutDataTypeStr=uint8
  Column_1(1B) : Outport
  Column_2(1B) : Outport  Port=2
  Column_3(1B) : Outport  Port=3
  Column_4(1B) : Outport  Port=4
  Column_5(1B) : Outport  Port=5
  Column_6(1B) : Outport  Port=6
  Column_7(1B) : Outport  Port=7
  Column_8(1B) : Outport  Port=8
  wires:
  Byte_05/1 -> Column_6(1B)/1
  Byte_04/1 -> Column_5(1B)/1
  Byte_01/1 -> Column_2(1B)/1
  Byte_07/1 -> Column_8(1B)/1
  Byte_03/1 -> Column_4(1B)/1
  Byte_06/1 -> Column_7(1B)/1
  Byte_1/1 -> Column_1(1B)/1
  Byte_02/1 -> Column_3(1B)/1

== system Pokus07_Display/Character_Table/Characters(ARROW_DOWN..RECTANGLE)2/Char_ARROW_DOWN ==
  Byte_01 : Constant  Value=char(2, ARROW_DOWN)  OutDataTypeStr=uint8
  Byte_02 : Constant  Value=char(3, ARROW_DOWN)  OutDataTypeStr=uint8
  Byte_03 : Constant  Value=char(4, ARROW_DOWN)  OutDataTypeStr=uint8
  Byte_04 : Constant  Value=char(5, ARROW_DOWN)  OutDataTypeStr=uint8
  Byte_05 : Constant  Value=char(6, ARROW_DOWN)  OutDataTypeStr=uint8
  Byte_06 : Constant  Value=char(7, ARROW_DOWN)  OutDataTypeStr=uint8
  Byte_07 : Constant  Value=char(8, ARROW_DOWN)  OutDataTypeStr=uint8
  Byte_1 : Constant  Value=char(1, ARROW_DOWN)  OutDataTypeStr=uint8
  Column_1(1B) : Outport
  Column_2(1B) : Outport  Port=2
  Column_3(1B) : Outport  Port=3
  Column_4(1B) : Outport  Port=4
  Column_5(1B) : Outport  Port=5
  Column_6(1B) : Outport  Port=6
  Column_7(1B) : Outport  Port=7
  Column_8(1B) : Outport  Port=8
  wires:
  Byte_05/1 -> Column_6(1B)/1
  Byte_04/1 -> Column_5(1B)/1
  Byte_01/1 -> Column_2(1B)/1
  Byte_07/1 -> Column_8(1B)/1
  Byte_03/1 -> Column_4(1B)/1
  Byte_06/1 -> Column_7(1B)/1
  Byte_1/1 -> Column_1(1B)/1
  Byte_02/1 -> Column_3(1B)/1

== system Pokus07_Display/Character_Table/Characters(ARROW_DOWN..RECTANGLE)2/Char_ARROW_LEFT ==
  Byte_01 : Constant  Value=char(2, ARROW_LEFT)  OutDataTypeStr=uint8
  Byte_02 : Constant  Value=char(3, ARROW_LEFT)  OutDataTypeStr=uint8
  Byte_03 : Constant  Value=char(4, ARROW_LEFT)  OutDataTypeStr=uint8
  Byte_04 : Constant  Value=char(5, ARROW_LEFT)  OutDataTypeStr=uint8
  Byte_05 : Constant  Value=char(6, ARROW_LEFT)  OutDataTypeStr=uint8
  Byte_06 : Constant  Value=char(7, ARROW_LEFT)  OutDataTypeStr=uint8
  Byte_07 : Constant  Value=char(8, ARROW_LEFT)  OutDataTypeStr=uint8
  Byte_1 : Constant  Value=char(1, ARROW_LEFT)  OutDataTypeStr=uint8
  Column_1(1B) : Outport
  Column_2(1B) : Outport  Port=2
  Column_3(1B) : Outport  Port=3
  Column_4(1B) : Outport  Port=4
  Column_5(1B) : Outport  Port=5
  Column_6(1B) : Outport  Port=6
  Column_7(1B) : Outport  Port=7
  Column_8(1B) : Outport  Port=8
  wires:
  Byte_05/1 -> Column_6(1B)/1
  Byte_04/1 -> Column_5(1B)/1
  Byte_01/1 -> Column_2(1B)/1
  Byte_07/1 -> Column_8(1B)/1
  Byte_03/1 -> Column_4(1B)/1
  Byte_06/1 -> Column_7(1B)/1
  Byte_1/1 -> Column_1(1B)/1
  Byte_02/1 -> Column_3(1B)/1

== system Pokus07_Display/Character_Table/Characters(ARROW_DOWN..RECTANGLE)2/Char_ARROW_RIGHT ==
  Byte_01 : Constant  Value=char(2, ARROW_RIGHT)  OutDataTypeStr=uint8
  Byte_02 : Constant  Value=char(3, ARROW_RIGHT)  OutDataTypeStr=uint8
  Byte_03 : Constant  Value=char(4, ARROW_RIGHT)  OutDataTypeStr=uint8
  Byte_04 : Constant  Value=char(5, ARROW_RIGHT)  OutDataTypeStr=uint8
  Byte_05 : Constant  Value=char(6, ARROW_RIGHT)  OutDataTypeStr=uint8
  Byte_06 : Constant  Value=char(7, ARROW_RIGHT)  OutDataTypeStr=uint8
  Byte_07 : Constant  Value=char(8, ARROW_RIGHT)  OutDataTypeStr=uint8
  Byte_1 : Constant  Value=char(1, ARROW_RIGHT)  OutDataTypeStr=uint8
  Column_1(1B) : Outport
  Column_2(1B) : Outport  Port=2
  Column_3(1B) : Outport  Port=3
  Column_4(1B) : Outport  Port=4
  Column_5(1B) : Outport  Port=5
  Column_6(1B) : Outport  Port=6
  Column_7(1B) : Outport  Port=7
  Column_8(1B) : Outport  Port=8
  wires:
  Byte_05/1 -> Column_6(1B)/1
  Byte_04/1 -> Column_5(1B)/1
  Byte_01/1 -> Column_2(1B)/1
  Byte_07/1 -> Column_8(1B)/1
  Byte_03/1 -> Column_4(1B)/1
  Byte_06/1 -> Column_7(1B)/1
  Byte_1/1 -> Column_1(1B)/1
  Byte_02/1 -> Column_3(1B)/1

== system Pokus07_Display/Character_Table/Characters(ARROW_DOWN..RECTANGLE)2/Char_COMMA ==
  Byte_01 : Constant  Value=char(2, COMMA)  OutDataTypeStr=uint8
  Byte_02 : Constant  Value=char(3, COMMA)  OutDataTypeStr=uint8
  Byte_03 : Constant  Value=char(4, COMMA)  OutDataTypeStr=uint8
  Byte_04 : Constant  Value=char(5, COMMA)  OutDataTypeStr=uint8
  Byte_05 : Constant  Value=char(6, COMMA)  OutDataTypeStr=uint8
  Byte_06 : Constant  Value=char(7, COMMA)  OutDataTypeStr=uint8
  Byte_07 : Constant  Value=char(8, COMMA)  OutDataTypeStr=uint8
  Byte_1 : Constant  Value=char(1, COMMA)  OutDataTypeStr=uint8
  Column_1(1B) : Outport
  Column_2(1B) : Outport  Port=2
  Column_3(1B) : Outport  Port=3
  Column_4(1B) : Outport  Port=4
  Column_5(1B) : Outport  Port=5
  Column_6(1B) : Outport  Port=6
  Column_7(1B) : Outport  Port=7
  Column_8(1B) : Outport  Port=8
  wires:
  Byte_05/1 -> Column_6(1B)/1
  Byte_04/1 -> Column_5(1B)/1
  Byte_01/1 -> Column_2(1B)/1
  Byte_07/1 -> Column_8(1B)/1
  Byte_03/1 -> Column_4(1B)/1
  Byte_06/1 -> Column_7(1B)/1
  Byte_1/1 -> Column_1(1B)/1
  Byte_02/1 -> Column_3(1B)/1

== system Pokus07_Display/Character_Table/Characters(ARROW_DOWN..RECTANGLE)2/Char_CURSOR ==
  Byte_01 : Constant  Value=char(2, CURSOR)  OutDataTypeStr=uint8
  Byte_02 : Constant  Value=char(3, CURSOR)  OutDataTypeStr=uint8
  Byte_03 : Constant  Value=char(4, CURSOR)  OutDataTypeStr=uint8
  Byte_04 : Constant  Value=char(5, CURSOR)  OutDataTypeStr=uint8
  Byte_05 : Constant  Value=char(6, CURSOR)  OutDataTypeStr=uint8
  Byte_06 : Constant  Value=char(7, CURSOR)  OutDataTypeStr=uint8
  Byte_07 : Constant  Value=char(8, CURSOR)  OutDataTypeStr=uint8
  Byte_1 : Constant  Value=char(1, CURSOR)  OutDataTypeStr=uint8
  Column_1(1B) : Outport
  Column_2(1B) : Outport  Port=2
  Column_3(1B) : Outport  Port=3
  Column_4(1B) : Outport  Port=4
  Column_5(1B) : Outport  Port=5
  Column_6(1B) : Outport  Port=6
  Column_7(1B) : Outport  Port=7
  Column_8(1B) : Outport  Port=8
  wires:
  Byte_05/1 -> Column_6(1B)/1
  Byte_04/1 -> Column_5(1B)/1
  Byte_01/1 -> Column_2(1B)/1
  Byte_07/1 -> Column_8(1B)/1
  Byte_03/1 -> Column_4(1B)/1
  Byte_06/1 -> Column_7(1B)/1
  Byte_1/1 -> Column_1(1B)/1
  Byte_02/1 -> Column_3(1B)/1

== system Pokus07_Display/Character_Table/Characters(ARROW_DOWN..RECTANGLE)2/Char_DOT ==
  Byte_01 : Constant  Value=char(2, DOT)  OutDataTypeStr=uint8
  Byte_02 : Constant  Value=char(3, DOT)  OutDataTypeStr=uint8
  Byte_03 : Constant  Value=char(4, DOT)  OutDataTypeStr=uint8
  Byte_04 : Constant  Value=char(5, DOT)  OutDataTypeStr=uint8
  Byte_05 : Constant  Value=char(6, DOT)  OutDataTypeStr=uint8
  Byte_06 : Constant  Value=char(7, DOT)  OutDataTypeStr=uint8
  Byte_07 : Constant  Value=char(8, DOT)  OutDataTypeStr=uint8
  Byte_1 : Constant  Value=char(1, DOT)  OutDataTypeStr=uint8
  Column_1(1B) : Outport
  Column_2(1B) : Outport  Port=2
  Column_3(1B) : Outport  Port=3
  Column_4(1B) : Outport  Port=4
  Column_5(1B) : Outport  Port=5
  Column_6(1B) : Outport  Port=6
  Column_7(1B) : Outport  Port=7
  Column_8(1B) : Outport  Port=8
  wires:
  Byte_05/1 -> Column_6(1B)/1
  Byte_04/1 -> Column_5(1B)/1
  Byte_01/1 -> Column_2(1B)/1
  Byte_07/1 -> Column_8(1B)/1
  Byte_03/1 -> Column_4(1B)/1
  Byte_06/1 -> Column_7(1B)/1
  Byte_1/1 -> Column_1(1B)/1
  Byte_02/1 -> Column_3(1B)/1

== system Pokus07_Display/Character_Table/Characters(ARROW_DOWN..RECTANGLE)2/Char_EXCLAMATION_MARK ==
  Byte_01 : Constant  Value=char(2, EXCLAMATION_MARK)  OutDataTypeStr=uint8
  Byte_02 : Constant  Value=char(3, EXCLAMATION_MARK)  OutDataTypeStr=uint8
  Byte_03 : Constant  Value=char(4, EXCLAMATION_MARK)  OutDataTypeStr=uint8
  Byte_04 : Constant  Value=char(5, EXCLAMATION_MARK)  OutDataTypeStr=uint8
  Byte_05 : Constant  Value=char(6, EXCLAMATION_MARK)  OutDataTypeStr=uint8
  Byte_06 : Constant  Value=char(7, EXCLAMATION_MARK)  OutDataTypeStr=uint8
  Byte_07 : Constant  Value=char(8, EXCLAMATION_MARK)  OutDataTypeStr=uint8
  Byte_1 : Constant  Value=char(1, EXCLAMATION_MARK)  OutDataTypeStr=uint8
  Column_1(1B) : Outport
  Column_2(1B) : Outport  Port=2
  Column_3(1B) : Outport  Port=3
  Column_4(1B) : Outport  Port=4
  Column_5(1B) : Outport  Port=5
  Column_6(1B) : Outport  Port=6
  Column_7(1B) : Outport  Port=7
  Column_8(1B) : Outport  Port=8
  wires:
  Byte_05/1 -> Column_6(1B)/1
  Byte_04/1 -> Column_5(1B)/1
  Byte_01/1 -> Column_2(1B)/1
  Byte_07/1 -> Column_8(1B)/1
  Byte_03/1 -> Column_4(1B)/1
  Byte_06/1 -> Column_7(1B)/1
  Byte_1/1 -> Column_1(1B)/1
  Byte_02/1 -> Column_3(1B)/1

== system Pokus07_Display/Character_Table/Characters(ARROW_DOWN..RECTANGLE)2/Char_LEFT_PARENTHESES ==
  Byte_01 : Constant  Value=char(2, LEFT_PARENTHESES)  OutDataTypeStr=uint8
  Byte_02 : Constant  Value=char(3, LEFT_PARENTHESES)  OutDataTypeStr=uint8
  Byte_03 : Constant  Value=char(4, LEFT_PARENTHESES)  OutDataTypeStr=uint8
  Byte_04 : Constant  Value=char(5, LEFT_PARENTHESES)  OutDataTypeStr=uint8
  Byte_05 : Constant  Value=char(6, LEFT_PARENTHESES)  OutDataTypeStr=uint8
  Byte_06 : Constant  Value=char(7, LEFT_PARENTHESES)  OutDataTypeStr=uint8
  Byte_07 : Constant  Value=char(8, LEFT_PARENTHESES)  OutDataTypeStr=uint8
  Byte_1 : Constant  Value=char(1, LEFT_PARENTHESES)  OutDataTypeStr=uint8
  Column_1(1B) : Outport
  Column_2(1B) : Outport  Port=2
  Column_3(1B) : Outport  Port=3
  Column_4(1B) : Outport  Port=4
  Column_5(1B) : Outport  Port=5
  Column_6(1B) : Outport  Port=6
  Column_7(1B) : Outport  Port=7
  Column_8(1B) : Outport  Port=8
  wires:
  Byte_05/1 -> Column_6(1B)/1
  Byte_04/1 -> Column_5(1B)/1
  Byte_01/1 -> Column_2(1B)/1
  Byte_07/1 -> Column_8(1B)/1
  Byte_03/1 -> Column_4(1B)/1
  Byte_06/1 -> Column_7(1B)/1
  Byte_1/1 -> Column_1(1B)/1
  Byte_02/1 -> Column_3(1B)/1

== system Pokus07_Display/Character_Table/Characters(ARROW_DOWN..RECTANGLE)2/Char_PERCENT ==
  Byte_01 : Constant  Value=char(2, PERCENT)  OutDataTypeStr=uint8
  Byte_02 : Constant  Value=char(3, PERCENT)  OutDataTypeStr=uint8
  Byte_03 : Constant  Value=char(4, PERCENT)  OutDataTypeStr=uint8
  Byte_04 : Constant  Value=char(5, PERCENT)  OutDataTypeStr=uint8
  Byte_05 : Constant  Value=char(6, PERCENT)  OutDataTypeStr=uint8
  Byte_06 : Constant  Value=char(7, PERCENT)  OutDataTypeStr=uint8
  Byte_07 : Constant  Value=char(8, PERCENT)  OutDataTypeStr=uint8
  Byte_1 : Constant  Value=char(1, PERCENT)  OutDataTypeStr=uint8
  Column_1(1B) : Outport
  Column_2(1B) : Outport  Port=2
  Column_3(1B) : Outport  Port=3
  Column_4(1B) : Outport  Port=4
  Column_5(1B) : Outport  Port=5
  Column_6(1B) : Outport  Port=6
  Column_7(1B) : Outport  Port=7
  Column_8(1B) : Outport  Port=8
  wires:
  Byte_05/1 -> Column_6(1B)/1
  Byte_04/1 -> Column_5(1B)/1
  Byte_01/1 -> Column_2(1B)/1
  Byte_07/1 -> Column_8(1B)/1
  Byte_03/1 -> Column_4(1B)/1
  Byte_06/1 -> Column_7(1B)/1
  Byte_1/1 -> Column_1(1B)/1
  Byte_02/1 -> Column_3(1B)/1

== system Pokus07_Display/Character_Table/Characters(ARROW_DOWN..RECTANGLE)2/Char_QUESTION_MARK ==
  Byte_01 : Constant  Value=char(2, QUESTION_MARK)  OutDataTypeStr=uint8
  Byte_02 : Constant  Value=char(3, QUESTION_MARK)  OutDataTypeStr=uint8
  Byte_03 : Constant  Value=char(4, QUESTION_MARK)  OutDataTypeStr=uint8
  Byte_04 : Constant  Value=char(5, QUESTION_MARK)  OutDataTypeStr=uint8
  Byte_05 : Constant  Value=char(6, QUESTION_MARK)  OutDataTypeStr=uint8
  Byte_06 : Constant  Value=char(7, QUESTION_MARK)  OutDataTypeStr=uint8
  Byte_07 : Constant  Value=char(8, QUESTION_MARK)  OutDataTypeStr=uint8
  Byte_1 : Constant  Value=char(1, QUESTION_MARK)  OutDataTypeStr=uint8
  Column_1(1B) : Outport
  Column_2(1B) : Outport  Port=2
  Column_3(1B) : Outport  Port=3
  Column_4(1B) : Outport  Port=4
  Column_5(1B) : Outport  Port=5
  Column_6(1B) : Outport  Port=6
  Column_7(1B) : Outport  Port=7
  Column_8(1B) : Outport  Port=8
  wires:
  Byte_05/1 -> Column_6(1B)/1
  Byte_04/1 -> Column_5(1B)/1
  Byte_01/1 -> Column_2(1B)/1
  Byte_07/1 -> Column_8(1B)/1
  Byte_03/1 -> Column_4(1B)/1
  Byte_06/1 -> Column_7(1B)/1
  Byte_1/1 -> Column_1(1B)/1
  Byte_02/1 -> Column_3(1B)/1

== system Pokus07_Display/Character_Table/Characters(ARROW_DOWN..RECTANGLE)2/Char_QUOTE ==
  Byte_01 : Constant  Value=char(2, QUOTE)  OutDataTypeStr=uint8
  Byte_02 : Constant  Value=char(3, QUOTE)  OutDataTypeStr=uint8
  Byte_03 : Constant  Value=char(4, QUOTE)  OutDataTypeStr=uint8
  Byte_04 : Constant  Value=char(5, QUOTE)  OutDataTypeStr=uint8
  Byte_05 : Constant  Value=char(6, QUOTE)  OutDataTypeStr=uint8
  Byte_06 : Constant  Value=char(7, QUOTE)  OutDataTypeStr=uint8
  Byte_07 : Constant  Value=char(8, QUOTE)  OutDataTypeStr=uint8
  Byte_1 : Constant  Value=char(1, QUOTE)  OutDataTypeStr=uint8
  Column_1(1B) : Outport
  Column_2(1B) : Outport  Port=2
  Column_3(1B) : Outport  Port=3
  Column_4(1B) : Outport  Port=4
  Column_5(1B) : Outport  Port=5
  Column_6(1B) : Outport  Port=6
  Column_7(1B) : Outport  Port=7
  Column_8(1B) : Outport  Port=8
  wires:
  Byte_05/1 -> Column_6(1B)/1
  Byte_04/1 -> Column_5(1B)/1
  Byte_01/1 -> Column_2(1B)/1
  Byte_07/1 -> Column_8(1B)/1
  Byte_03/1 -> Column_4(1B)/1
  Byte_06/1 -> Column_7(1B)/1
  Byte_1/1 -> Column_1(1B)/1
  Byte_02/1 -> Column_3(1B)/1
